simulink model "PalmSat"  (R2017b)
settings: Solver=VariableStepAuto  StartTime=0.0  StopTime=10  RelTol=1e-3
values from neighbouring files (symbols this model uses):
  Bm = Kt*I/2200    (= 0.0113875331796)    [PalmSatModelScript.m]
  Br = Bm    (= 0.0113875331796)    [PalmSatModelScript.m]
  Jm = 16307/10^9    (= 1.6307e-05)    [PalmSatModelScript.m]
  Jr = 163076/10^9    (= 0.000163076)    [PalmSatModelScript.m]
  K = 0.002    [PalmSatModelScript.m]
  Kt = Kw/0.00684    (= 25.0525729951)    [PalmSatModelScript.m]
  Kw = 60*2*pi/2200    (= 0.171359599287)    [PalmSatModelScript.m]
  La = 74.4*10^-6    (= 7.44e-05)    [PalmSatModelScript.m]
  Ra = 0.225    [PalmSatModelScript.m]
undefined symbols (not defined in the file or in its folder): IA, IB, IC
settings Model: Creator=Gpiaia  LastModifiedBy=Gpiaia

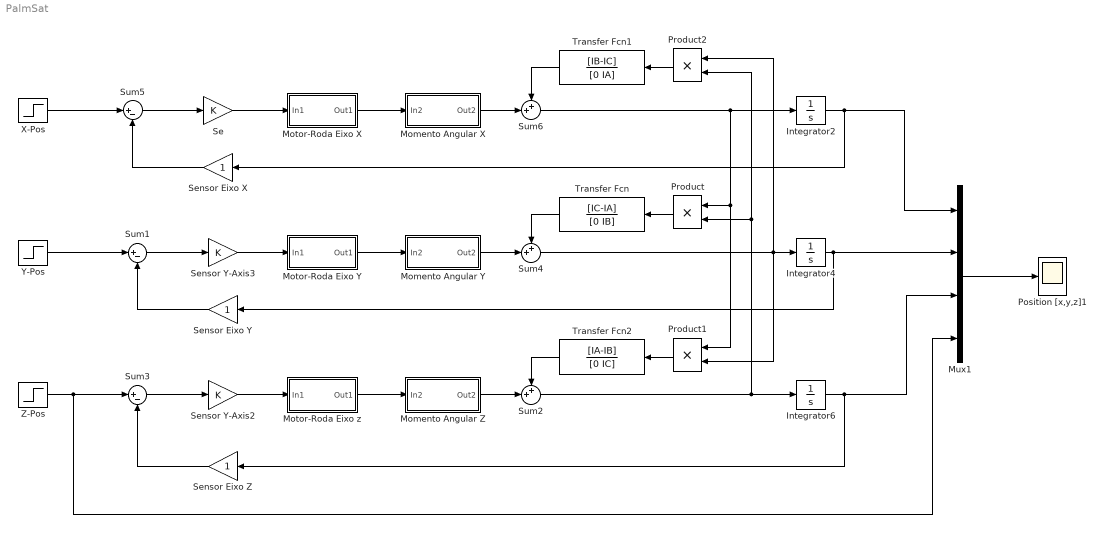
== system PalmSat ==
  Integrator2 : Integrator
  Integrator4 : Integrator
  Integrator6 : Integrator
  Momento Angular X : Subsystem
  Momento Angular Y : Subsystem
  Momento Angular Z : Subsystem
  Motor-Roda Eixo X : Subsystem
  Motor-Roda Eixo Y : Subsystem
  Motor-Roda Eixo z : Subsystem
  Mux1 : Mux
  Position [x,y,z]1 : Scope
  Product : Product
  Product1 : Product
  Product2 : Product
  Se : Gain  Gain=K
  Sensor Eixo X : Gain
  Sensor Eixo Y : Gain
  Sensor Eixo Z : Gain
  Sensor Y-Axis2 : Gain  Gain=K
  Sensor Y-Axis3 : Gain  Gain=K
  Sum1 : Sum  Inputs=|+-
  Sum2 : Sum  Inputs=++|
  Sum3 : Sum  Inputs=|+-
  Sum4 : Sum  Inputs=++|
  Sum5 : Sum  Inputs=|+-
  Sum6 : Sum  Inputs=++|
  Transfer Fcn : TransferFcn  Numerator=[IC-IA]  Denominator=[0 IB]
  Transfer Fcn1 : TransferFcn  Numerator=[IB-IC]  Denominator=[0 IA]
  Transfer Fcn2 : TransferFcn  Numerator=[IA-IB]  Denominator=[0 IC]
  X-Pos : Step  Time=5  After=0  SampleTime=0
  Y-Pos : Step  Time=0  After=0  SampleTime=0
  Z-Pos : Step  After=45  SampleTime=0
  wires:
  Momento Angular X/1(Out2) -> Sum6/2
  Product1/1 -> Transfer Fcn2/1
  Product2/1 -> Transfer Fcn1/1
  Motor-Roda Eixo Y/1(Out1) -> Momento Angular Y/1(In2)
  Z-Pos/1 -> Mux1/4, Sum3/1
  Sensor Y-Axis2/1 -> Motor-Roda Eixo z/1(In1)
  Sensor Eixo Y/1 -> Sum1/2
  Mux1/1 -> Position [x,y,z]1/1
  Sum5/1 -> Se/1
  Sensor Y-Axis3/1 -> Motor-Roda Eixo Y/1(In1)
  Sensor Eixo Z/1 -> Sum3/2
  Se/1 -> Motor-Roda Eixo X/1(In1)
  Momento Angular Y/1(Out2) -> Sum4/2
  Sum6/1 -> Integrator2/1, Product1/1, Product/1
  Sensor Eixo X/1 -> Sum5/2
  Transfer Fcn/1 -> Sum4/1
  Product/1 -> Transfer Fcn/1
  Sum4/1 -> Product1/2, Product2/1, Integrator4/1
  Integrator4/1 -> Sensor Eixo Y/1, Mux1/2
  Integrator6/1 -> Mux1/3, Sensor Eixo Z/1
  Motor-Roda Eixo X/1(Out1) -> Momento Angular X/1(In2)
  Transfer Fcn2/1 -> Sum2/1
  Integrator2/1 -> Sensor Eixo X/1, Mux1/1
  Sum3/1 -> Sensor Y-Axis2/1
  Sum1/1 -> Sensor Y-Axis3/1
  Sum2/1 -> Product2/2, Product/2, Integrator6/1
  Transfer Fcn1/1 -> Sum6/1
  X-Pos/1 -> Sum5/1
  Y-Pos/1 -> Sum1/1
  Motor-Roda Eixo z/1(Out1) -> Momento Angular Z/1(In2)
  Momento Angular Z/1(Out2) -> Sum2/2

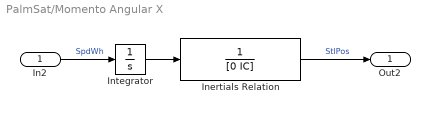
== system PalmSat/Momento Angular X ==
  In2 : Inport
  Inertials Relation : TransferFcn  Numerator=[0 1]  Denominator=[0 IC]
  Integrator : Integrator
  Out2 : Outport
  wires:
  In2/1 -> Integrator/1  "SpdWh"
  Inertials Relation/1 -> Out2/1  "StlPos"
  Integrator/1 -> Inertials Relation/1

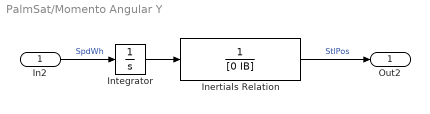
== system PalmSat/Momento Angular Y ==
  In2 : Inport
  Inertials Relation : TransferFcn  Numerator=[0 1]  Denominator=[0 IB]
  Integrator : Integrator
  Out2 : Outport
  wires:
  In2/1 -> Integrator/1  "SpdWh"
  Inertials Relation/1 -> Out2/1  "StlPos"
  Integrator/1 -> Inertials Relation/1

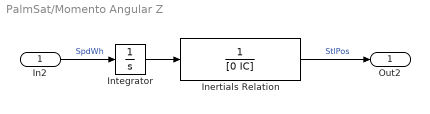
== system PalmSat/Momento Angular Z ==
  In2 : Inport
  Inertials Relation : TransferFcn  Numerator=[0 1]  Denominator=[0 IC]
  Integrator : Integrator
  Out2 : Outport
  wires:
  In2/1 -> Integrator/1  "SpdWh"
  Inertials Relation/1 -> Out2/1  "StlPos"
  Integrator/1 -> Inertials Relation/1

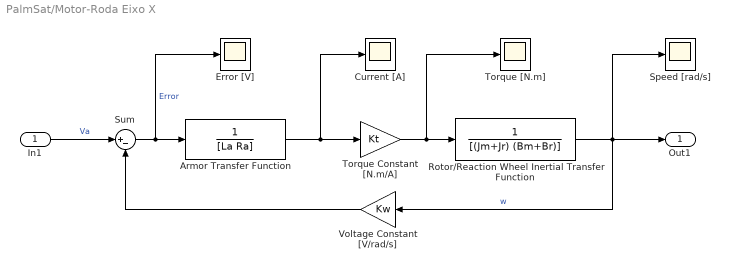
== system PalmSat/Motor-Roda Eixo X ==
  In1 : Inport
  Armor Transfer Function : TransferFcn  Denominator=[La Ra]
  Current [A] : Scope
  Error [V] : Scope
  Rotor/Reaction Wheel Inertial Transfer Function : TransferFcn  Denominator=[(Jm+Jr) (Bm+Br)]
  Speed [rad/s] : Scope
  Sum : Sum  Inputs=|+-
  Torque [N.m] : Scope
  Torque Constant [N.m/A] : Gain  Gain=Kt
  Voltage Constant [V/rad/s] : Gain  Gain=Kw
  Out1 : Outport
  wires:
  Armor Transfer Function/1 -> Current [A]/1, Torque Constant [N.m/A]/1
  Rotor/Reaction Wheel Inertial Transfer Function/1 -> Out1/1, Voltage Constant [V/rad/s]/1, Speed [rad/s]/1  "w"
  In1/1 -> Sum/1  "Va"
  Torque Constant [N.m/A]/1 -> Rotor/Reaction Wheel Inertial Transfer Function/1, Torque [N.m]/1
  Voltage Constant [V/rad/s]/1 -> Sum/2
  Sum/1 -> Error [V]/1, Armor Transfer Function/1  "Error"

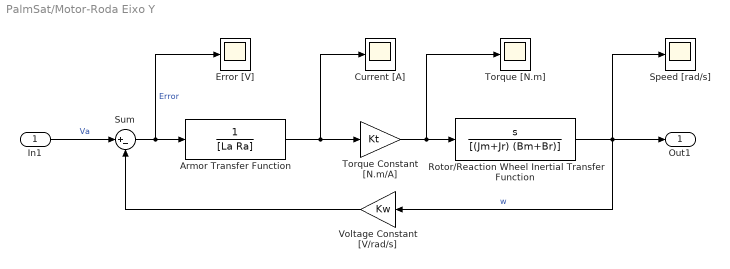
== system PalmSat/Motor-Roda Eixo Y ==
  In1 : Inport
  Armor Transfer Function : TransferFcn  Denominator=[La Ra]
  Current [A] : Scope
  Error [V] : Scope
  Rotor/Reaction Wheel Inertial Transfer Function : TransferFcn  Numerator=[1 0]  Denominator=[(Jm+Jr) (Bm+Br)]
  Speed [rad/s] : Scope
  Sum : Sum  Inputs=|+-
  Torque [N.m] : Scope
  Torque Constant [N.m/A] : Gain  Gain=Kt
  Voltage Constant [V/rad/s] : Gain  Gain=Kw
  Out1 : Outport
  wires:
  Armor Transfer Function/1 -> Current [A]/1, Torque Constant [N.m/A]/1
  Rotor/Reaction Wheel Inertial Transfer Function/1 -> Out1/1, Voltage Constant [V/rad/s]/1, Speed [rad/s]/1  "w"
  In1/1 -> Sum/1  "Va"
  Torque Constant [N.m/A]/1 -> Rotor/Reaction Wheel Inertial Transfer Function/1, Torque [N.m]/1
  Voltage Constant [V/rad/s]/1 -> Sum/2
  Sum/1 -> Error [V]/1, Armor Transfer Function/1  "Error"

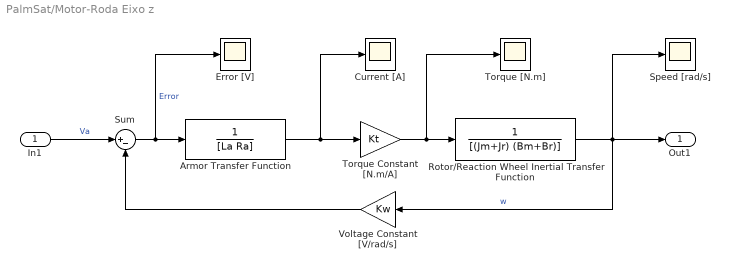
== system PalmSat/Motor-Roda Eixo z ==
  In1 : Inport
  Armor Transfer Function : TransferFcn  Denominator=[La Ra]
  Current [A] : Scope
  Error [V] : Scope
  Rotor/Reaction Wheel Inertial Transfer Function : TransferFcn  Denominator=[(Jm+Jr) (Bm+Br)]
  Speed [rad/s] : Scope
  Sum : Sum  Inputs=|+-
  Torque [N.m] : Scope
  Torque Constant [N.m/A] : Gain  Gain=Kt
  Voltage Constant [V/rad/s] : Gain  Gain=Kw
  Out1 : Outport
  wires:
  Armor Transfer Function/1 -> Current [A]/1, Torque Constant [N.m/A]/1
  Rotor/Reaction Wheel Inertial Transfer Function/1 -> Out1/1, Voltage Constant [V/rad/s]/1, Speed [rad/s]/1  "w"
  In1/1 -> Sum/1  "Va"
  Torque Constant [N.m/A]/1 -> Rotor/Reaction Wheel Inertial Transfer Function/1, Torque [N.m]/1
  Voltage Constant [V/rad/s]/1 -> Sum/2
  Sum/1 -> Error [V]/1, Armor Transfer Function/1  "Error"
